simulink model "cm_test"  (R2015a)
settings: Solver=ode45  StartTime=0.0  StopTime=inf  MaxStep=1e-3  RelTol=1e-3
values from neighbouring files (symbols this model uses):
  ctr_law = struct    [Parameters.m]
  IMU = struct    [Parameters.m]
  lateral_control = true    [Parameters.m]
  longit_control = true    [Parameters.m]
  low_ctr = struct    [Parameters.m]
  mag = struct    [Parameters.m]
  steer_flag = 0    [Parameters.m]
  steer_sensor = struct    [Parameters.m]
  vhcl = struct    [Parameters.m]
undefined symbols (not defined in the file or in its folder): odo
libraries: CarMaker4SL x29, dspquant2 x6, simulink x1, aerolibtransform2 x1
(part 2 of 2)

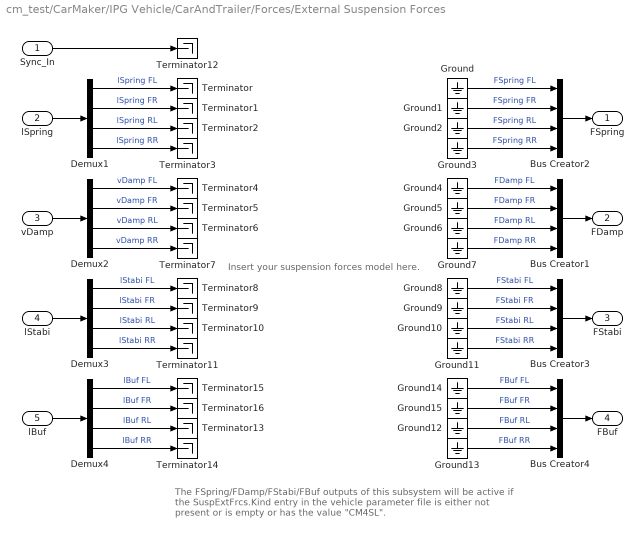
== system cm_test/CarMaker/IPG Vehicle/CarAndTrailer/Forces/External Suspension Forces ==
  note: The FSpring/FDamp/FStabi/FBuf outputs of this subsystem will be
      | active if the SuspExtFrcs.Kind entry in the vehicle parameter file
      | is either not present or is empty or has the value "CM4SL".
  note: Insert your suspension forces model here.
  Sync_In : Inport
  lSpring : Inport  Port=2
  vDamp : Inport  Port=3
  lStabi : Inport  Port=4
  lBuf : Inport  Port=5
  Bus Creator{1..4} (4 alike) : BusCreator
  Demux{1..4} (4 alike) : Demux
  Ground{,1..15} (16 alike) : Ground
  Terminator{,1..16} (17 alike) : Terminator
  FSpring : Outport
  FDamp : Outport  Port=2
  FStabi : Outport  Port=3
  FBuf : Outport  Port=4
  wires:
  lBuf/1 -> Demux4/1
  Demux4/1 -> Terminator15/1  "lBuf FL"
  Demux4/2 -> Terminator16/1  "lBuf FR"
  Demux4/3 -> Terminator13/1  "lBuf RL"
  Demux4/4 -> Terminator14/1  "lBuf RR"
  Ground14/1 -> Bus Creator4/1  "FBuf FL"
  Ground15/1 -> Bus Creator4/2  "FBuf FR"
  Ground12/1 -> Bus Creator4/3  "FBuf RL"
  Ground13/1 -> Bus Creator4/4  "FBuf RR"
  Bus Creator4/1 -> FBuf/1
  Sync_In/1 -> Terminator12/1
  lSpring/1 -> Demux1/1
  vDamp/1 -> Demux2/1
  lStabi/1 -> Demux3/1
  Demux3/1 -> Terminator8/1  "lStabi FL"
  Demux3/2 -> Terminator9/1  "lStabi FR"
  Demux3/3 -> Terminator10/1  "lStabi RL"
  Demux3/4 -> Terminator11/1  "lStabi RR"
  Demux1/1 -> Terminator/1  "lSpring FL"
  Demux1/2 -> Terminator1/1  "lSpring FR"
  Demux1/3 -> Terminator2/1  "lSpring RL"
  Demux1/4 -> Terminator3/1  "lSpring RR"
  Demux2/1 -> Terminator4/1  "vDamp FL"
  Demux2/2 -> Terminator5/1  "vDamp FR"
  Demux2/3 -> Terminator6/1  "vDamp RL"
  Demux2/4 -> Terminator7/1  "vDamp RR"
  Bus Creator2/1 -> FSpring/1
  Ground/1 -> Bus Creator2/1  "FSpring FL"
  Ground1/1 -> Bus Creator2/2  "FSpring FR"
  Ground2/1 -> Bus Creator2/3  "FSpring RL"
  Ground3/1 -> Bus Creator2/4  "FSpring RR"
  Ground4/1 -> Bus Creator1/1  "FDamp FL"
  Ground5/1 -> Bus Creator1/2  "FDamp FR"
  Ground6/1 -> Bus Creator1/3  "FDamp RL"
  Ground7/1 -> Bus Creator1/4  "FDamp RR"
  Bus Creator1/1 -> FDamp/1
  Ground8/1 -> Bus Creator3/1  "FStabi FL"
  Ground9/1 -> Bus Creator3/2  "FStabi FR"
  Ground10/1 -> Bus Creator3/3  "FStabi RL"
  Ground11/1 -> Bus Creator3/4  "FStabi RR"
  Bus Creator3/1 -> FStabi/1

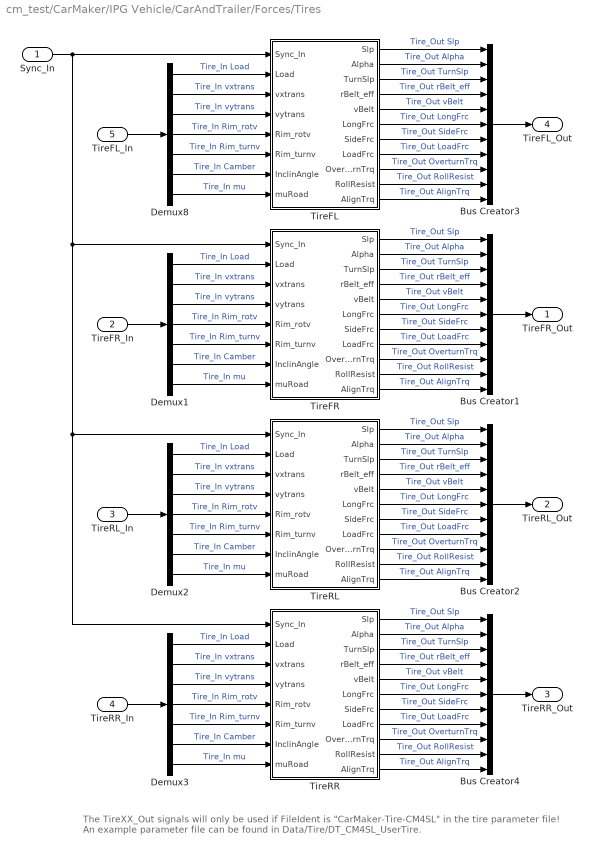
== system cm_test/CarMaker/IPG Vehicle/CarAndTrailer/Forces/Tires ==
  note: The TireXX_Out signals will only be used if FileIdent is "CarMaker-Tire-CM4SL" in the tire parameter file!
      | An example parameter file can be found in Data/Tire/DT_CM4SL_UserTire.
  Sync_In : Inport
  TireFR_In : Inport  Port=2
  TireRL_In : Inport  Port=3
  TireRR_In : Inport  Port=4
  TireFL_In : Inport  Port=5
  Bus Creator{1..4} (4 alike) : BusCreator  Inputs=11
  Demux{1..3,8} (4 alike) : Demux  Outputs=7
  TireFL : Subsystem
  TireFR : Subsystem
  TireRL : Subsystem
  TireRR : Subsystem
  TireFR_Out : Outport
  TireRL_Out : Outport  Port=2
  TireRR_Out : Outport  Port=3
  TireFL_Out : Outport  Port=4
  wires:
  Sync_In/1 -> TireRR/1(Sync_In), TireRL/1(Sync_In), TireFR/1(Sync_In), TireFL/1(Sync_In)
  Bus Creator4/1 -> TireRR_Out/1
  Bus Creator2/1 -> TireRL_Out/1
  Bus Creator1/1 -> TireFR_Out/1
  Demux3/5 -> TireRR/6(Rim_turnv)  "Tire_In Rim_turnv"
  Demux3/4 -> TireRR/5(Rim_rotv)  "Tire_In Rim_rotv"
  Demux3/1 -> TireRR/2(Load)  "Tire_In Load"
  Demux3/7 -> TireRR/8(muRoad)  "Tire_In mu"
  Demux3/6 -> TireRR/7(InclinAngle)  "Tire_In Camber"
  Demux3/2 -> TireRR/3(vxtrans)  "Tire_In vxtrans"
  Demux3/3 -> TireRR/4(vytrans)  "Tire_In vytrans"
  TireRR/11(AlignTrq) -> Bus Creator4/11  "Tire_Out AlignTrq"
  TireRR/10(RollResist) -> Bus Creator4/10  "Tire_Out RollResist"
  TireRR/9(OverturnTrq) -> Bus Creator4/9  "Tire_Out OverturnTrq"
  TireRR/8(LoadFrc) -> Bus Creator4/8  "Tire_Out LoadFrc"
  TireRR/7(SideFrc) -> Bus Creator4/7  "Tire_Out SideFrc"
  TireRR/6(LongFrc) -> Bus Creator4/6  "Tire_Out LongFrc"
  TireRR/5(vBelt) -> Bus Creator4/5  "Tire_Out vBelt"
  TireRR/4(rBelt_eff) -> Bus Creator4/4  "Tire_Out rBelt_eff"
  TireRR/3(TurnSlp) -> Bus Creator4/3  "Tire_Out TurnSlp"
  TireRR/1(Slp) -> Bus Creator4/1  "Tire_Out Slp"
  TireRR/2(Alpha) -> Bus Creator4/2  "Tire_Out Alpha"
  Demux2/5 -> TireRL/6(Rim_turnv)  "Tire_In Rim_turnv"
  Demux2/4 -> TireRL/5(Rim_rotv)  "Tire_In Rim_rotv"
  Demux2/1 -> TireRL/2(Load)  "Tire_In Load"
  Demux2/7 -> TireRL/8(muRoad)  "Tire_In mu"
  Demux2/6 -> TireRL/7(InclinAngle)  "Tire_In Camber"
  Demux2/2 -> TireRL/3(vxtrans)  "Tire_In vxtrans"
  Demux2/3 -> TireRL/4(vytrans)  "Tire_In vytrans"
  TireRL/11(AlignTrq) -> Bus Creator2/11  "Tire_Out AlignTrq"
  TireRL/10(RollResist) -> Bus Creator2/10  "Tire_Out RollResist"
  TireRL/9(OverturnTrq) -> Bus Creator2/9  "Tire_Out OverturnTrq"
  TireRL/8(LoadFrc) -> Bus Creator2/8  "Tire_Out LoadFrc"
  TireRL/7(SideFrc) -> Bus Creator2/7  "Tire_Out SideFrc"
  TireRL/6(LongFrc) -> Bus Creator2/6  "Tire_Out LongFrc"
  TireRL/5(vBelt) -> Bus Creator2/5  "Tire_Out vBelt"
  TireRL/4(rBelt_eff) -> Bus Creator2/4  "Tire_Out rBelt_eff"
  TireRL/3(TurnSlp) -> Bus Creator2/3  "Tire_Out TurnSlp"
  TireRL/1(Slp) -> Bus Creator2/1  "Tire_Out Slp"
  TireRL/2(Alpha) -> Bus Creator2/2  "Tire_Out Alpha"
  Demux1/5 -> TireFR/6(Rim_turnv)  "Tire_In Rim_turnv"
  Demux1/4 -> TireFR/5(Rim_rotv)  "Tire_In Rim_rotv"
  Demux1/1 -> TireFR/2(Load)  "Tire_In Load"
  Demux1/7 -> TireFR/8(muRoad)  "Tire_In mu"
  Demux1/6 -> TireFR/7(InclinAngle)  "Tire_In Camber"
  Demux1/2 -> TireFR/3(vxtrans)  "Tire_In vxtrans"
  Demux1/3 -> TireFR/4(vytrans)  "Tire_In vytrans"
  TireFR/11(AlignTrq) -> Bus Creator1/11  "Tire_Out AlignTrq"
  TireFR/10(RollResist) -> Bus Creator1/10  "Tire_Out RollResist"
  TireFR/9(OverturnTrq) -> Bus Creator1/9  "Tire_Out OverturnTrq"
  TireFR/8(LoadFrc) -> Bus Creator1/8  "Tire_Out LoadFrc"
  TireFR/7(SideFrc) -> Bus Creator1/7  "Tire_Out SideFrc"
  TireFR/6(LongFrc) -> Bus Creator1/6  "Tire_Out LongFrc"
  TireFR/5(vBelt) -> Bus Creator1/5  "Tire_Out vBelt"
  TireFR/4(rBelt_eff) -> Bus Creator1/4  "Tire_Out rBelt_eff"
  TireFR/3(TurnSlp) -> Bus Creator1/3  "Tire_Out TurnSlp"
  TireFR/1(Slp) -> Bus Creator1/1  "Tire_Out Slp"
  TireFR/2(Alpha) -> Bus Creator1/2  "Tire_Out Alpha"
  Demux8/5 -> TireFL/6(Rim_turnv)  "Tire_In Rim_turnv"
  Demux8/4 -> TireFL/5(Rim_rotv)  "Tire_In Rim_rotv"
  TireFL_In/1 -> Demux8/1
  Demux8/1 -> TireFL/2(Load)  "Tire_In Load"
  Demux8/7 -> TireFL/8(muRoad)  "Tire_In mu"
  Demux8/6 -> TireFL/7(InclinAngle)  "Tire_In Camber"
  Demux8/2 -> TireFL/3(vxtrans)  "Tire_In vxtrans"
  Demux8/3 -> TireFL/4(vytrans)  "Tire_In vytrans"
  TireFL/11(AlignTrq) -> Bus Creator3/11  "Tire_Out AlignTrq"
  TireFL/10(RollResist) -> Bus Creator3/10  "Tire_Out RollResist"
  TireFL/9(OverturnTrq) -> Bus Creator3/9  "Tire_Out OverturnTrq"
  TireFL/8(LoadFrc) -> Bus Creator3/8  "Tire_Out LoadFrc"
  TireFL/7(SideFrc) -> Bus Creator3/7  "Tire_Out SideFrc"
  TireFL/6(LongFrc) -> Bus Creator3/6  "Tire_Out LongFrc"
  TireFL/5(vBelt) -> Bus Creator3/5  "Tire_Out vBelt"
  TireFL/4(rBelt_eff) -> Bus Creator3/4  "Tire_Out rBelt_eff"
  TireFL/3(TurnSlp) -> Bus Creator3/3  "Tire_Out TurnSlp"
  TireFL/1(Slp) -> Bus Creator3/1  "Tire_Out Slp"
  TireFL/2(Alpha) -> Bus Creator3/2  "Tire_Out Alpha"
  Bus Creator3/1 -> TireFL_Out/1
  TireFR_In/1 -> Demux1/1
  TireRL_In/1 -> Demux2/1
  TireRR_In/1 -> Demux3/1

== system cm_test/CarMaker/IPG Vehicle/CarAndTrailer/Forces/Vehicle Forces ==
  Sync_In : Inport
  Bus Creator1 : BusCreator  Inputs=12
  Bus Creator5 : BusCreator  Inputs=13
  Bus Creator8 : BusCreator  Inputs=16
  Demux : Demux  Outputs=16
  Demux1 : Demux  Outputs=12
  Demux5 : Demux  Outputs=13
  Forces : S-Function  FunctionName=CM_Sfun  Parameters='Forces'
  Sync_Out : Outport
  Car.Virtual : Outport  Port=2
  Car.Aero : Outport  Port=3
  Car.Load : Outport  Port=4
  wires:
  Demux/16 -> Bus Creator8/16  "Car Load_3 tz"
  Demux/15 -> Bus Creator8/15  "Car Load_3 ty"
  Demux/14 -> Bus Creator8/14  "Car Load_3 tx"
  Demux/13 -> Bus Creator8/13  "Car Load_3 mass"
  Demux1/12 -> Bus Creator1/12  "Car Virtual Trq_0 z"
  Demux1/11 -> Bus Creator1/11  "Car Virtual Trq_0 y"
  Demux1/10 -> Bus Creator1/10  "Car Virtual Trq_0 x"
  Demux1/9 -> Bus Creator1/9  "Car Virtual Trq_1 z"
  Demux1/8 -> Bus Creator1/8  "Car Virtual Trq_1 y"
  Demux1/7 -> Bus Creator1/7  "Car Virtual Trq_1 x"
  Demux1/6 -> Bus Creator1/6  "Car Virtual Frc_0 z"
  Demux1/5 -> Bus Creator1/5  "Car Virtual Frc_0 y"
  Demux1/4 -> Bus Creator1/4  "Car Virtual Frc_0 x"
  Sync_In/1 -> Forces/1
  Forces/1 -> Sync_Out/1
  Bus Creator5/1 -> Car.Aero/1
  Demux1/1 -> Bus Creator1/1  "Car Virtual Frc_1 x"
  Demux1/2 -> Bus Creator1/2  "Car Virtual Frc_1 y"
  Demux1/3 -> Bus Creator1/3  "Car Virtual Frc_1 z"
  Forces/3 -> Demux5/1
  Forces/2 -> Demux1/1
  Bus Creator1/1 -> Car.Virtual/1
  Bus Creator8/1 -> Car.Load/1
  Demux/1 -> Bus Creator8/1  "Car Load_0 mass"
  Demux/2 -> Bus Creator8/2  "Car Load_0 tx"
  Demux/3 -> Bus Creator8/3  "Car Load_0 ty"
  Demux/4 -> Bus Creator8/4  "Car Load_0 tz"
  Demux/5 -> Bus Creator8/5  "Car Load_1 mass"
  Demux/6 -> Bus Creator8/6  "Car Load_1 tx"
  Demux/7 -> Bus Creator8/7  "Car Load_1 ty"
  Demux/8 -> Bus Creator8/8  "Car Load_1 tz"
  Demux/9 -> Bus Creator8/9  "Car Load_2 mass"
  Demux/10 -> Bus Creator8/10  "Car Load_2 tx"
  Demux/11 -> Bus Creator8/11  "Car Load_2 ty"
  Demux/12 -> Bus Creator8/12  "Car Load_2 tz"
  Forces/4 -> Demux/1
  Demux5/11 -> Bus Creator5/11  "car Aero Trq_1 x"
  Demux5/12 -> Bus Creator5/12  "car Aero Trq_1 y"
  Demux5/13 -> Bus Creator5/13  "car Aero Trq_1 z"
  Demux5/10 -> Bus Creator5/10  "car Aero Frc_1 z"
  Demux5/9 -> Bus Creator5/9  "car Aero Frc_1 y"
  Demux5/8 -> Bus Creator5/8  "car Aero Frc_1 x"
  Demux5/1 -> Bus Creator5/1  "Vehicle sRoadAero"
  Demux5/2 -> Bus Creator5/2  "Vehicle Wind_vel_0 x"
  Demux5/3 -> Bus Creator5/3  "Vehicle Wind_vel_0 y"
  Demux5/4 -> Bus Creator5/4  "Vehicle Wind_vel_0 z"
  Demux5/5 -> Bus Creator5/5  "car Aero vRes_1 x"
  Demux5/6 -> Bus Creator5/6  "car Aero vRes_1 y"
  Demux5/7 -> Bus Creator5/7  "car Aero vRes_1 z"

== system cm_test/CarMaker/IPG Vehicle/CarAndTrailer/Trailer/CreateBus Car.Hitch.FrcTrq ==
  In1 : Inport
  Bus Creator7 : BusCreator  Inputs=6
  Demux7 : Demux  Outputs=6
  Car.Hitch.FrcTrq : Outport
  wires:
  In1/1 -> Demux7/1
  Bus Creator7/1 -> Car.Hitch.FrcTrq/1
  Demux7/6 -> Bus Creator7/6  "Car Hitch Trq2Car z"
  Demux7/5 -> Bus Creator7/5  "Car Hitch Trq2Car y"
  Demux7/4 -> Bus Creator7/4  "Car Hitch Trq2Car x"
  Demux7/3 -> Bus Creator7/3  "Car Hitch Frc2Car z"
  Demux7/2 -> Bus Creator7/2  "Car Hitch Frc2Car y"
  Demux7/1 -> Bus Creator7/1  "Car Hitch Frc2Car x"

== system cm_test/CarMaker/IPG Vehicle/CarAndTrailer/Trailer/CreateBus Vhcl.Motion ==
  In1 : Inport
  Demux1 : Demux  Outputs=16
  Mux1 : Mux  Inputs=16
  Out1 : Outport
  wires:
  Demux1/1 -> Mux1/1  "Vhcl v"
  Demux1/2 -> Mux1/2  "Vhcl Distance"
  Demux1/3 -> Mux1/3  "Vhcl sRoad"
  Demux1/4 -> Mux1/4  "Vhcl sRoadAero"
  Demux1/5 -> Mux1/5  "Vhcl Hitch_Pos x"
  Demux1/6 -> Mux1/6  "Vhcl Hitch_Pos y"
  Demux1/7 -> Mux1/7  "Vhcl Hitch_Pos z"
  Demux1/8 -> Mux1/8  "Vhcl Roll"
  Demux1/9 -> Mux1/9  "Vhcl RollVel"
  Demux1/10 -> Mux1/10  "Vhcl RollAcc"
  Demux1/11 -> Mux1/11  "Vhcl Pitch"
  Demux1/12 -> Mux1/12  "Vhcl PitchVel"
  Demux1/13 -> Mux1/13  "Vhcl PitchAcc"
  Demux1/14 -> Mux1/14  "Vhcl Yaw"
  Demux1/15 -> Mux1/15  "Vhcl YawRate"
  Demux1/16 -> Mux1/16  "Vhcl YawAcc"
  In1/1 -> Demux1/1
  Mux1/1 -> Out1/1

== system cm_test/CarMaker/IPG Vehicle/CarAndTrailer/Trailer/CreateBus Vhcl.PoI ==
  In1 : Inport
  Bus Creator3 : BusCreator  Inputs=18
  Demux3 : Demux  Outputs=18
  Out1 : Outport
  wires:
  Demux3/18 -> Bus Creator3/18  "Vhcl PoI_GCS Elev"
  Demux3/17 -> Bus Creator3/17  "Vhcl PoI_GCS Lat"
  Demux3/16 -> Bus Creator3/16  "Vhcl PoI_GCS Long"
  Demux3/15 -> Bus Creator3/15  "Vhcl PoI_Acc_1 z"
  Demux3/14 -> Bus Creator3/14  "Vhcl PoI_Acc_1 y"
  Demux3/13 -> Bus Creator3/13  "Vhcl PoI_Acc_1 x"
  Demux3/12 -> Bus Creator3/12  "Vhcl PoI_Vel_1 z"
  Demux3/11 -> Bus Creator3/11  "Vhcl PoI_Vel_1 y"
  Demux3/10 -> Bus Creator3/10  "Vhcl PoI_Vel_1 x"
  Demux3/9 -> Bus Creator3/9  "Vhcl PoI_Acc z"
  Demux3/8 -> Bus Creator3/8  "Vhcl PoI_Acc y"
  Demux3/7 -> Bus Creator3/7  "Vhcl PoI_Acc x"
  Demux3/6 -> Bus Creator3/6  "Vhcl PoI_Vel z"
  Demux3/5 -> Bus Creator3/5  "Vhcl PoI_Vel y"
  Demux3/4 -> Bus Creator3/4  "Vhcl PoI_Vel x"
  Demux3/3 -> Bus Creator3/3  "Vhcl PoI_Pos z"
  Demux3/2 -> Bus Creator3/2  "Vhcl PoI_Pos y"
  In1/1 -> Demux3/1
  Bus Creator3/1 -> Out1/1
  Demux3/1 -> Bus Creator3/1  "Vhcl PoI_Pos x"

== system cm_test/CarMaker/IPG Vehicle/CarAndTrailer/Trailer/CreateBus Vhcl.Steering ==
  In1 : Inport
  Bus Creator3 : BusCreator
  Demux : Demux
  Out1 : Outport
  wires:
  Bus Creator3/1 -> Out1/1
  Demux/1 -> Bus Creator3/1  "Vhcl Steering Ang"
  Demux/3 -> Bus Creator3/3  "Vhcl Steering AngAcc"
  Demux/2 -> Bus Creator3/2  "Vhcl Steering AngVel"
  Demux/4 -> Bus Creator3/4  "Vhcl Steering Trq"
  In1/1 -> Demux/1

== system cm_test/CarMaker/IPG Vehicle/CarAndTrailer/Trailer/CreateBus Vhcl.Wheel.FL ==
  In1 : Inport
  Bus Creator3 : BusCreator  Inputs=14
  Demux3 : Demux  Outputs=14
  Out1 : Outport
  wires:
  Demux3/14 -> Bus Creator3/14  "Vhcl Wheel FL Trq_WhlBearing"
  Demux3/13 -> Bus Creator3/13  "Vhcl Wheel FL Trq_T2W"
  Demux3/12 -> Bus Creator3/12  "Vhcl Wheel FL SideSlip"
  Demux3/11 -> Bus Creator3/11  "Vhcl Wheel FL LongSlip"
  Demux3/10 -> Bus Creator3/10  "Vhcl Wheel FL vBelt"
  Demux3/9 -> Bus Creator3/9  "Vhcl Wheel FL Fz"
  Demux3/8 -> Bus Creator3/8  "Vhcl Wheel FL Fy"
  Demux3/7 -> Bus Creator3/7  "Vhcl Wheel FL Fx"
  Demux3/6 -> Bus Creator3/6  "Vhcl Wheel FL r_zxy z"
  Demux3/5 -> Bus Creator3/5  "Vhcl Wheel FL r_zxy y"
  Demux3/4 -> Bus Creator3/4  "Vhcl Wheel FL r_zxy x"
  Demux3/3 -> Bus Creator3/3  "Vhcl Wheel FL t z"
  Demux3/2 -> Bus Creator3/2  "Vhcl Wheel FL t y"
  In1/1 -> Demux3/1
  Bus Creator3/1 -> Out1/1
  Demux3/1 -> Bus Creator3/1  "Vhcl Wheel FL t x"

== system cm_test/CarMaker/IPG Vehicle/CarAndTrailer/Trailer/CreateBus Vhcl.Wheel.FR ==
  In1 : Inport
  Bus Creator3 : BusCreator  Inputs=14
  Demux3 : Demux  Outputs=14
  Out1 : Outport
  wires:
  Demux3/14 -> Bus Creator3/14  "Vhcl Wheel FR Trq_WhlBearing"
  Demux3/13 -> Bus Creator3/13  "Vhcl Wheel FR Trq_T2W"
  Demux3/12 -> Bus Creator3/12  "Vhcl Wheel FR SideSlip"
  Demux3/11 -> Bus Creator3/11  "Vhcl Wheel FR LongSlip"
  Demux3/10 -> Bus Creator3/10  "Vhcl Wheel FR vBelt"
  Demux3/9 -> Bus Creator3/9  "Vhcl Wheel FR Fz"
  Demux3/8 -> Bus Creator3/8  "Vhcl Wheel FR Fy"
  Demux3/7 -> Bus Creator3/7  "Vhcl Wheel FR Fx"
  Demux3/6 -> Bus Creator3/6  "Vhcl Wheel FR r_zxy z"
  Demux3/5 -> Bus Creator3/5  "Vhcl Wheel FR r_zxy y"
  Demux3/4 -> Bus Creator3/4  "Vhcl Wheel FR r_zxy x"
  Demux3/3 -> Bus Creator3/3  "Vhcl Wheel FR t z"
  Demux3/2 -> Bus Creator3/2  "Vhcl Wheel FR t y"
  In1/1 -> Demux3/1
  Bus Creator3/1 -> Out1/1
  Demux3/1 -> Bus Creator3/1  "Vhcl Wheel FR t x"

== system cm_test/CarMaker/IPG Vehicle/CarAndTrailer/Trailer/CreateBus Vhcl.Wheel.RL ==
  In1 : Inport
  Bus Creator3 : BusCreator  Inputs=14
  Demux3 : Demux  Outputs=14
  Out1 : Outport
  wires:
  Demux3/14 -> Bus Creator3/14  "Vhcl Wheel RL Trq_WhlBearing"
  Demux3/13 -> Bus Creator3/13  "Vhcl Wheel RL Trq_T2W"
  Demux3/12 -> Bus Creator3/12  "Vhcl Wheel RL SideSlip"
  Demux3/11 -> Bus Creator3/11  "Vhcl Wheel RL LongSlip"
  Demux3/10 -> Bus Creator3/10  "Vhcl Wheel RL vBelt"
  Demux3/9 -> Bus Creator3/9  "Vhcl Wheel RL Fz"
  Demux3/8 -> Bus Creator3/8  "Vhcl Wheel RL Fy"
  Demux3/7 -> Bus Creator3/7  "Vhcl Wheel RL Fx"
  Demux3/6 -> Bus Creator3/6  "Vhcl Wheel RL r_zxy z"
  Demux3/5 -> Bus Creator3/5  "Vhcl Wheel RL r_zxy y"
  Demux3/4 -> Bus Creator3/4  "Vhcl Wheel RL r_zxy x"
  Demux3/3 -> Bus Creator3/3  "Vhcl Wheel RL t z"
  Demux3/2 -> Bus Creator3/2  "Vhcl Wheel RL t y"
  In1/1 -> Demux3/1
  Bus Creator3/1 -> Out1/1
  Demux3/1 -> Bus Creator3/1  "Vhcl Wheel RL t x"

== system cm_test/CarMaker/IPG Vehicle/CarAndTrailer/Trailer/CreateBus Vhcl.Wheel.RR ==
  In1 : Inport
  Bus Creator3 : BusCreator  Inputs=14
  Demux3 : Demux  Outputs=14
  Out1 : Outport
  wires:
  Demux3/14 -> Bus Creator3/14  "Vhcl Wheel RR Trq_WhlBearing"
  Demux3/13 -> Bus Creator3/13  "Vhcl Wheel RR Trq_T2W"
  Demux3/12 -> Bus Creator3/12  "Vhcl Wheel RR SideSlip"
  Demux3/11 -> Bus Creator3/11  "Vhcl Wheel RR LongSlip"
  Demux3/10 -> Bus Creator3/10  "Vhcl Wheel RR vBelt"
  Demux3/9 -> Bus Creator3/9  "Vhcl Wheel RR Fz"
  Demux3/8 -> Bus Creator3/8  "Vhcl Wheel RR Fy"
  Demux3/7 -> Bus Creator3/7  "Vhcl Wheel RR Fx"
  Demux3/6 -> Bus Creator3/6  "Vhcl Wheel RR r_zxy z"
  Demux3/5 -> Bus Creator3/5  "Vhcl Wheel RR r_zxy y"
  Demux3/4 -> Bus Creator3/4  "Vhcl Wheel RR r_zxy x"
  Demux3/3 -> Bus Creator3/3  "Vhcl Wheel RR t z"
  Demux3/2 -> Bus Creator3/2  "Vhcl Wheel RR t y"
  In1/1 -> Demux3/1
  Bus Creator3/1 -> Out1/1
  Demux3/1 -> Bus Creator3/1  "Vhcl Wheel RR t x"

== system cm_test/CarMaker/VehicleControl/Sensors/IMU/Accelerometers ==
  Mux : Mux  Inputs=3
  Read Alpha.x : CarMaker4SL/Read CM Dict  xname=BodySensor.BD00.Alpha_0.x  xsync=off
  Read Alpha.y : CarMaker4SL/Read CM Dict  xname=BodySensor.BD00.Alpha_0.y  xsync=off
  Read Alpha.z : CarMaker4SL/Read CM Dict  xname=BodySensor.BD00.Alpha_0.z  xsync=off
  Scope : Scope
  Scope1 : Scope
  Scope2 : Scope
  accels_out : Outport
  wires:
  Read Alpha.y/1 -> Scope1/1, Mux/2
  Read Alpha.x/1 -> Scope/1, Mux/1
  Read Alpha.z/1 -> Scope2/1, Mux/3
  Mux/1 -> accels_out/1

== system cm_test/CarMaker/VehicleControl/Sensors/IMU/Gyroscopes ==
  Mux : Mux  Inputs=3
  Read Omega.x : CarMaker4SL/Read CM Dict  xname=BodySensor.BD00.Omega_0.x  xsync=off
  Read Omega.y : CarMaker4SL/Read CM Dict  xname=BodySensor.BD00.Omega_0.y  xsync=off
  Read Omega.z : CarMaker4SL/Read CM Dict  xname=BodySensor.BD00.Omega_0.z  xsync=off
  Scope : Scope
      settings: YMin=-10  YMax=10
  Scope1 : Scope
  Scope2 : Scope
  gyros_out : Outport
  wires:
  Read Omega.y/1 -> Scope1/1, Mux/2
  Read Omega.x/1 -> Scope/1, Mux/1
  Read Omega.z/1 -> Scope2/1, Mux/3
  Mux/1 -> gyros_out/1

== system cm_test/CarMaker/VehicleControl/Sensors/RPSensor/Preview pt pos in Fr1 ==
  Display{,1..3} (4 alike) : Display
  MatProduct : Product  Multiplication=Matrix(*)
  Rotation Angles to Direction Cosine Matrix : aerolibtransform2/Rotation Angles to Direction Cosine Matrix  rotationOrder=ZYX
  car rotation in Fr0 : Subsystem
  preview pt pos in Fr0 with car origin as origin of Fr0 : Subsystem
  prev_pt_pos_Fr1 : Outport
  wires:
  Rotation Angles to Direction Cosine Matrix/1 -> Display1/1, MatProduct/1
  preview pt pos in Fr0 with car origin as origin of Fr0/1(prev_pt_pos_Fr0) -> Display3/1, MatProduct/2  "prev_pt_pos_Fr0"
  car rotation in Fr0/1(3D_angle) -> Display/1, Rotation Angles to Direction Cosine Matrix/1
  MatProduct/1 -> Display2/1, prev_pt_pos_Fr1/1  "prev_pt_pos_Fr1"

== system cm_test/CarMaker/VehicleControl/Sensors/Steering angle (rad)/Mean of 2 values ==
  vec : Inport
  Add : Sum
  Demux : Demux  Outputs=2
  Gain : Gain  Gain=0.5
  mean : Outport
  wires:
  Add/1 -> Gain/1
  Gain/1 -> mean/1
  Demux/2 -> Add/2
  Demux/1 -> Add/1
  vec/1 -> Demux/1

== system cm_test/CarMaker/VehicleControl/Sensors/odometry/Mean of 2 values ==
  vec : Inport
  Add : Sum
  Demux : Demux  Outputs=2
  Gain : Gain  Gain=0.5
  mean : Outport
  wires:
  Add/1 -> Gain/1
  Gain/1 -> mean/1
  Demux/2 -> Add/2
  Demux/1 -> Add/1
  vec/1 -> Demux/1

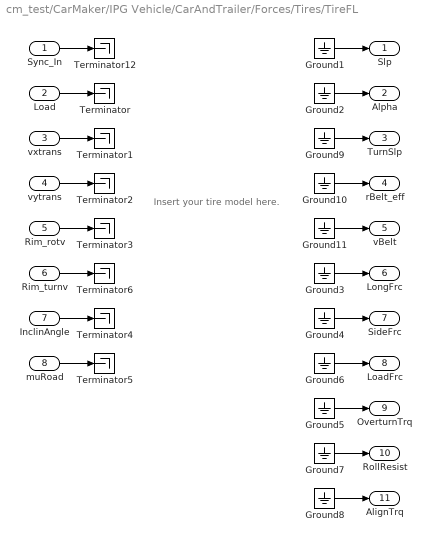
== system cm_test/CarMaker/IPG Vehicle/CarAndTrailer/Forces/Tires/TireFL ==
  note: Insert your tire model here.
  Sync_In : Inport
  Load : Inport  Port=2
  vxtrans : Inport  Port=3
  vytrans : Inport  Port=4
  Rim_rotv : Inport  Port=5
  Rim_turnv : Inport  Port=6
  InclinAngle : Inport  Port=7
  muRoad : Inport  Port=8
  Ground{1..11} (11 alike) : Ground
  Terminator{,1..6,12} (8 alike) : Terminator
  Slp : Outport
  Alpha : Outport  Port=2
  TurnSlp : Outport  Port=3
  rBelt_eff : Outport  Port=4
  vBelt : Outport  Port=5
  LongFrc : Outport  Port=6
  SideFrc : Outport  Port=7
  LoadFrc : Outport  Port=8
  OverturnTrq : Outport  Port=9
  RollResist : Outport  Port=10
  AlignTrq : Outport  Port=11
  wires:
  Ground11/1 -> vBelt/1
  Ground10/1 -> rBelt_eff/1
  Ground9/1 -> TurnSlp/1
  Rim_turnv/1 -> Terminator6/1
  Sync_In/1 -> Terminator12/1
  Ground2/1 -> Alpha/1
  Ground3/1 -> LongFrc/1
  Ground4/1 -> SideFrc/1
  Ground5/1 -> OverturnTrq/1
  vxtrans/1 -> Terminator1/1
  vytrans/1 -> Terminator2/1
  Rim_rotv/1 -> Terminator3/1
  InclinAngle/1 -> Terminator4/1
  muRoad/1 -> Terminator5/1
  Load/1 -> Terminator/1
  Ground1/1 -> Slp/1
  Ground6/1 -> LoadFrc/1
  Ground7/1 -> RollResist/1
  Ground8/1 -> AlignTrq/1

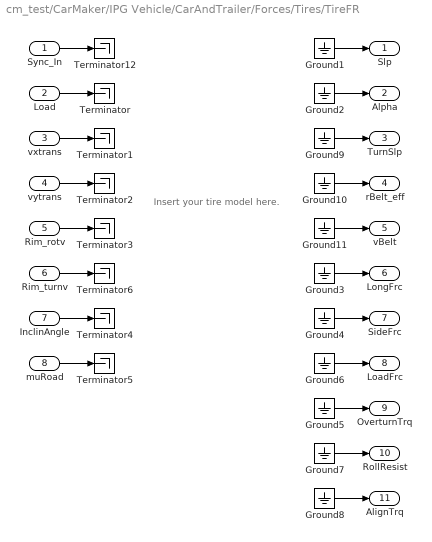
== system cm_test/CarMaker/IPG Vehicle/CarAndTrailer/Forces/Tires/TireFR ==
  note: Insert your tire model here.
  Sync_In : Inport
  Load : Inport  Port=2
  vxtrans : Inport  Port=3
  vytrans : Inport  Port=4
  Rim_rotv : Inport  Port=5
  Rim_turnv : Inport  Port=6
  InclinAngle : Inport  Port=7
  muRoad : Inport  Port=8
  Ground{1..11} (11 alike) : Ground
  Terminator{,1..6,12} (8 alike) : Terminator
  Slp : Outport
  Alpha : Outport  Port=2
  TurnSlp : Outport  Port=3
  rBelt_eff : Outport  Port=4
  vBelt : Outport  Port=5
  LongFrc : Outport  Port=6
  SideFrc : Outport  Port=7
  LoadFrc : Outport  Port=8
  OverturnTrq : Outport  Port=9
  RollResist : Outport  Port=10
  AlignTrq : Outport  Port=11
  wires:
  Ground11/1 -> vBelt/1
  Ground10/1 -> rBelt_eff/1
  Ground9/1 -> TurnSlp/1
  Rim_turnv/1 -> Terminator6/1
  Sync_In/1 -> Terminator12/1
  Ground2/1 -> Alpha/1
  Ground3/1 -> LongFrc/1
  Ground4/1 -> SideFrc/1
  Ground5/1 -> OverturnTrq/1
  vxtrans/1 -> Terminator1/1
  vytrans/1 -> Terminator2/1
  Rim_rotv/1 -> Terminator3/1
  InclinAngle/1 -> Terminator4/1
  muRoad/1 -> Terminator5/1
  Load/1 -> Terminator/1
  Ground1/1 -> Slp/1
  Ground6/1 -> LoadFrc/1
  Ground7/1 -> RollResist/1
  Ground8/1 -> AlignTrq/1

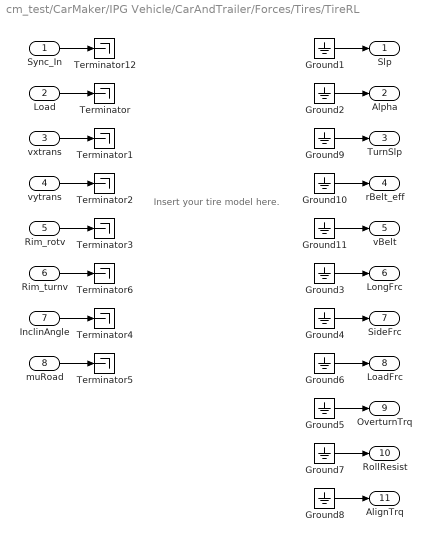
== system cm_test/CarMaker/IPG Vehicle/CarAndTrailer/Forces/Tires/TireRL ==
  note: Insert your tire model here.
  Sync_In : Inport
  Load : Inport  Port=2
  vxtrans : Inport  Port=3
  vytrans : Inport  Port=4
  Rim_rotv : Inport  Port=5
  Rim_turnv : Inport  Port=6
  InclinAngle : Inport  Port=7
  muRoad : Inport  Port=8
  Ground{1..11} (11 alike) : Ground
  Terminator{,1..6,12} (8 alike) : Terminator
  Slp : Outport
  Alpha : Outport  Port=2
  TurnSlp : Outport  Port=3
  rBelt_eff : Outport  Port=4
  vBelt : Outport  Port=5
  LongFrc : Outport  Port=6
  SideFrc : Outport  Port=7
  LoadFrc : Outport  Port=8
  OverturnTrq : Outport  Port=9
  RollResist : Outport  Port=10
  AlignTrq : Outport  Port=11
  wires:
  Ground11/1 -> vBelt/1
  Ground10/1 -> rBelt_eff/1
  Ground9/1 -> TurnSlp/1
  Rim_turnv/1 -> Terminator6/1
  Sync_In/1 -> Terminator12/1
  Ground2/1 -> Alpha/1
  Ground3/1 -> LongFrc/1
  Ground4/1 -> SideFrc/1
  Ground5/1 -> OverturnTrq/1
  vxtrans/1 -> Terminator1/1
  vytrans/1 -> Terminator2/1
  Rim_rotv/1 -> Terminator3/1
  InclinAngle/1 -> Terminator4/1
  muRoad/1 -> Terminator5/1
  Load/1 -> Terminator/1
  Ground1/1 -> Slp/1
  Ground6/1 -> LoadFrc/1
  Ground7/1 -> RollResist/1
  Ground8/1 -> AlignTrq/1

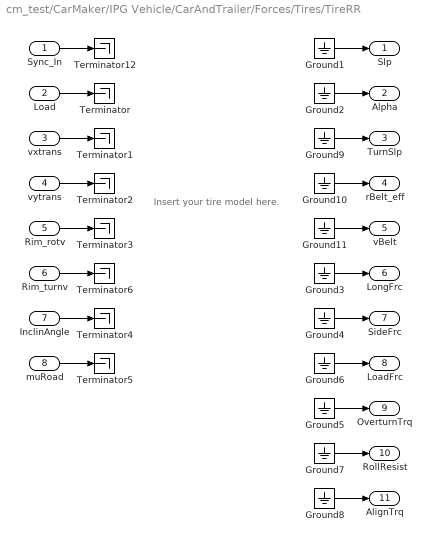
== system cm_test/CarMaker/IPG Vehicle/CarAndTrailer/Forces/Tires/TireRR ==
  note: Insert your tire model here.
  Sync_In : Inport
  Load : Inport  Port=2
  vxtrans : Inport  Port=3
  vytrans : Inport  Port=4
  Rim_rotv : Inport  Port=5
  Rim_turnv : Inport  Port=6
  InclinAngle : Inport  Port=7
  muRoad : Inport  Port=8
  Ground{1..11} (11 alike) : Ground
  Terminator{,1..6,12} (8 alike) : Terminator
  Slp : Outport
  Alpha : Outport  Port=2
  TurnSlp : Outport  Port=3
  rBelt_eff : Outport  Port=4
  vBelt : Outport  Port=5
  LongFrc : Outport  Port=6
  SideFrc : Outport  Port=7
  LoadFrc : Outport  Port=8
  OverturnTrq : Outport  Port=9
  RollResist : Outport  Port=10
  AlignTrq : Outport  Port=11
  wires:
  Ground11/1 -> vBelt/1
  Ground10/1 -> rBelt_eff/1
  Ground9/1 -> TurnSlp/1
  Rim_turnv/1 -> Terminator6/1
  Sync_In/1 -> Terminator12/1
  Ground2/1 -> Alpha/1
  Ground3/1 -> LongFrc/1
  Ground4/1 -> SideFrc/1
  Ground5/1 -> OverturnTrq/1
  vxtrans/1 -> Terminator1/1
  vytrans/1 -> Terminator2/1
  Rim_rotv/1 -> Terminator3/1
  InclinAngle/1 -> Terminator4/1
  muRoad/1 -> Terminator5/1
  Load/1 -> Terminator/1
  Ground1/1 -> Slp/1
  Ground6/1 -> LoadFrc/1
  Ground7/1 -> RollResist/1
  Ground8/1 -> AlignTrq/1

== system cm_test/CarMaker/VehicleControl/Sensors/RPSensor/Preview pt pos in Fr1/car rotation in Fr0 ==
  Mux : Mux  Inputs=3
  pitch angle : CarMaker4SL/Read CM Dict  xname=Vhcl.Pitch  xsync=off
  roll angle : CarMaker4SL/Read CM Dict  xname=Vhcl.Roll  xsync=off
  yaw angle : CarMaker4SL/Read CM Dict  xname=Vhcl.Yaw  xsync=off
  3D_angle : Outport
  wires:
  pitch angle/1 -> Mux/2
  roll angle/1 -> Mux/3
  yaw angle/1 -> Mux/1
  Mux/1 -> 3D_angle/1

== system cm_test/CarMaker/VehicleControl/Sensors/RPSensor/Preview pt pos in Fr1/preview pt pos in Fr0 with car origin as origin of Fr0 ==
  Display : Display
  Display1 : Display
  ground truth absolute pos of preview point : Subsystem
  ground truth absolute pos of vehicle origin (rear of vehicle) : Subsystem
  sub : Sum  Inputs=+-
  prev_pt_pos_Fr0 : Outport
  wires:
  sub/1 -> prev_pt_pos_Fr0/1
  ground truth absolute pos of vehicle origin (rear of vehicle)/1(vehicle_pos) -> Display1/1, sub/2
  ground truth absolute pos of preview point/1(preview_point_pos) -> Display/1, sub/1

== system cm_test/CarMaker/VehicleControl/Sensors/RPSensor/Preview pt pos in Fr1/preview pt pos in Fr0 with car origin as origin of Fr0/ground truth absolute pos of preview point ==
  Mux : Mux  Inputs=3
  Preview point absolute position : CarMaker4SL/Read CM Dict  xname=RPSensor.RP00.Path.tx  xsync=off
  Preview point absolute position1 : CarMaker4SL/Read CM Dict  xname=RPSensor.RP00.Path.ty  xsync=off
  Preview point absolute position2 : CarMaker4SL/Read CM Dict  xname=RPSensor.RP00.Path.tz  xsync=off
  preview_point_pos : Outport
  wires:
  Preview point absolute position/1 -> Mux/1
  Mux/1 -> preview_point_pos/1
  Preview point absolute position2/1 -> Mux/3
  Preview point absolute position1/1 -> Mux/2

== system cm_test/CarMaker/VehicleControl/Sensors/RPSensor/Preview pt pos in Fr1/preview pt pos in Fr0 with car origin as origin of Fr0/ground truth absolute pos of vehicle origin (rear of vehicle) ==
  Mux : Mux  Inputs=3
  Vehicle origin absolute position -x : CarMaker4SL/Read CM Dict  xname=Vhcl.Fr1.x  xsync=off
  Vehicle origin absolute position -y : CarMaker4SL/Read CM Dict  xname=Vhcl.Fr1.y  xsync=off
  Vehicle origin absolute position- z : CarMaker4SL/Read CM Dict  xname=Vhcl.Fr1.z  xsync=off
  vehicle_pos : Outport
  wires:
  Vehicle origin absolute position -x/1 -> Mux/1
  Vehicle origin absolute position -y/1 -> Mux/2
  Vehicle origin absolute position- z/1 -> Mux/3
  Mux/1 -> vehicle_pos/1

== matlab function cm_test/CarMaker/VehicleControl/Autonomous driving/low level controller ==
  data: sensors_in input; v_ref input; gamma_ref input; accel output; steer_flag input; low_ctr input; vhcl input; steer output
function [accel, steer] = fcn(sensors_in, v_ref, gamma_ref, steer_flag, ...
    low_ctr, vhcl)
%% Transforms output of control law into driver-like inputs for CM model
% implements low level controllers for steerign and speed and maps the
% outputs to be fed to CarMaker "VehicleControlUpd" model.
% 
% inputs:
% - target speed or acceleration
% - target steering angle (at front wheels)
%
% outputs:
% accel vector, composed of:
%   - brake
%   - gas
% steer vector composed of: 
%   - steering angle at steering wheel
%   - steering velocity at steering wheel
%   - steering accel at steering wheel
%   - steering torque at steering wheel
%
% depending on the steering mode, some of the steering signals might be set
% to zero.

%% Retrieves inputs and parameters

Fs = low_ctr.Fs;

% measures for feedback
% longitudinal acceleration
% a = sensors_in.imu_out.Alpha_0(1);
% actual speed
v = sensors_in.odo_out.vel_from_motor;

% wheel radius
R_wheel = vhcl.wheel_radius;

% vehicle mass
mass = vhcl.mass;

% mapping coeff for gas pedal (linear coeff only for the moment)
torque_to_gas = 1 ./ (low_ctr.trq_full - low_ctr.trq_zero);

% mapping for brake pedal
% vector of 2 coeffs: 1 for a front wheel and 1 for a rear wheel.
% to directly have the torque for an axle, the brake_to_Trq coeffs have
% been multiplied by 2.
torque_to_brake = 1 ./ (2*low_ctr.brake_to_Trq);

% steering angle to angle of steering wheel
steer_coeff = low_ctr.st_angle_to_st_wheel;

% CAREFUL: mappings for steering and brake are approximate. Need a proper
% control loop (along with smooth references) to ensure proper tracking.

%% Output initialization

steer_angle = 0;
steer_vel = 0;
steer_acc = 0;
steer_torque = 0;

accel = zeros(2,1);
steer = zeros(4,1);

% depending on the steering controller, either the 3 first or juste the
% last one will be filled.

%% Speed controller

Ts = 1/Fs;

% Converts desired speed into ref acceleration to get to that speed

% output acceleration (to be given to motor controller and it will do what
% it can)

% shaping controller, based on the error on speed. There is no feedback
% on acceleration yet
% the controller implemented is only proportional at the moment
a_ref_raw = low_ctr.K_accel * (v_ref - v) / Ts;

% saturation
a_ref = clip_signal(a_ref_raw, -low_ctr.max_accel, low_ctr.max_accel);


% TO IMPLEMENT LATER
% actual feedback loop on acceleration


%% Steering angle controller


% Angle steering ----------------
if steer_flag == 0;

    % shaping controller
    steer_ref = gamma_ref * steer_coeff;

    % feedback controller 
    % (not needed in this mode if we have a perfect mapping)
    steer_ref_fbk = steer_ref;

    % output
    steer_angle = steer_ref_fbk;


% Torque steering ----------------
elseif steer_flag == 1
    % only feedback for this one.

    % NOT IMPLEMENTED YET

end


%% Conversion of outputs

% accel to torque at wheels
torque_ref = mass * R_wheel * a_ref;

% gas pedal output
% torque at wheels to torque at engine (division by gear ratio)
torque_mot_ref = torque_ref / vhcl.gear_ratio;
% takes positive part of reference torque
gas_torque = clip_signal(torque_mot_ref, 0, inf);
% norms it with gas pedal to acceleration torque mapping
gas_out = gas_torque * torque_to_gas;
% clips to 1 (gas output is in [0;1])
gas_out_clipped = clip_signal(gas_out, 0, 1);

% brake pedal output
% takes negative part of reference torque and puts it in positive domain
% this is the TOTAL brake torque  at the wheels (sum on 4 wheels)
brake_torque = clip_signal(-torque_ref, 0, inf);
% norms it with gas pedal to acceleration torque mapping
% adds the two coeffs for each axle to be multiplied with the total torque
brake_out = brake_torque * sum(torque_to_brake);
% clips to 1 (brake output is in [0;1])
brake_out_clipped = clip_signal(brake_out, 0, 1);


%% Formatting of the outputs
% defines all bus variables for car control : gas/brake, lights, 
% blinkers, ... 

%
gas = gas_out_clipped;
brake = brake_out_clipped;


accel(1) = brake;
accel(2) = gas;

steer(1) = steer_angle;
steer(2) = steer_vel;
steer(3) = steer_acc;
steer(4) = steer_torque;


end



function x_clipped = clip_signal(x, lower_bnd, upper_bnd)
%%
%

x_clipped = max(lower_bnd, min(upper_bnd, x));

end

== matlab function cm_test/CarMaker/VehicleControl/Autonomous driving/trajectory tracking controller ==
  data: sensors_in input; v output; ctr_law input; vehicle input; gamma output; ctr_vars output
function [v, gamma, ctr_vars] = control_law(sensors_in, ctr_law, vehicle)
% input: "sensor_in", with the accessible fields:
% - imu_out
% - lat_errs
% - steer_angles
%
% fields of "sensors_in.imu_out" :
% - Omega_0 : gyro output on 3 axis in rad/s
% - Alpha_0 : accelerometers output on 3 
%
% fields of "lat_errs" :
% - lat_pos_ctr_road : 
% - lat_pos_ctr_lane :
% - hdg_err :
% - path_hdg :
% - curve_xy :
%
% fields of "steer_angles"
% - steer_angle_1 :
% - steer_angle_2 : 
% - mean_angle :

%% input retrieval


%% choice and application of control law

% markers for choosing the control law
Vilca_flag = ctr_law.flag == 1;
Stanley_flag = ctr_law.flag == 2;
Kinematic_flag = ctr_law.flag == 3;

if Vilca_flag
    % one term for the steering output has been deactivated
    [v, gamma, ctr_vars] = VilcaController(sensors_in, ctr_law, vehicle);
elseif Stanley_flag
    % Stanley's controller
    % NB; v is equal to the target speed specified in the parameters file.
    % This controller is not a speed controller.
    [v, gamma, ctr_vars] = StanleyController(sensors_in,...
        ctr_law, vehicle);
elseif Stanley_flag
    % Kinematic controller based on chained form
    [v, gamma, ctr_vars] = KinematicController(sensors_in, ctr_law, ...
        vehicle);
else
    v = 0;
    gamma = 0;
    ctr_vars = zeros(4,1);
end




end


function [v,gamma, ctr_vars] = ...
    VilcaController(sensors_in, ctr_law, vehicle)
%%
%

%% Control variables calculation

% target orientation in Fr0
% theta_T = sensors_in.rpsensor_out.path_hdg;

% angular error between vehicle direction and target direction
% DEBUG : "-" for correction of conventions
e_theta = - sensors_in(1).rpsensor_out.hdg_err;

% preview point pos wrt centre of rear axle
prev_pt_pos_r_axle = sensors_in(1).rpsensor_out.preview_pt_pos_Fr1 ...
    - [vehicle.rear_axle_x; 0; 0];
% x coordinate of target in Fr1 with rear axle as origin
e_x = prev_pt_pos_r_axle(1);
% y coordinate of target in Fr1 with rear axle as origin
e_y = prev_pt_pos_r_axle(2);
% absolute distance to target (preview point)
d = sqrt(e_x^2 + e_y^2);
% vehicle angular pos in target frame with reference direction being the
% direction of target but looking backwards
% is also:
% target heading - vehicle polar position in global frame as seen from
% target
% equation 3.13 of [Vilca2015]. The advantage is that it uses previously
% defined variables so if these ones are correct, the rest will also be.
e_RT = atan2(e_x*tan(e_theta)-e_y, e_x+tan(e_theta)*e_y);

% radius of curvature at target
r_ct = 1 / sensors_in(1).rpsensor_out.curve_xy; % careful if infinity
% target speed
% (projection of vehicle speed along path)
% in reality it's not ctr_law.target_speed because there will be a tracking
% error. The actual speed of the vehicle should be measured and projected
% on the path direction at the preview point
v_t = ctr_law.target_speed;
% pos of target in vehicle's frame


%% Parameters retrieval

% control law coeffs
% K_vec = zeros(1,6);
K_vec =  ctr_law.K_vilca;

K_d = K_vec(1);
K_l = K_vec(2);
K_o = K_vec(3);
K_x = K_vec(4);
K_RT = K_vec(5);
K_theta = K_vec(6);

% wheelbase
l_b = vehicle.wheelbase;

%% Pre-calculations

% CAUTION: the term with d^2 messes everything up. It is much bigger than
% the rest and leads to saturation.
c_c = 1 / (r_ct*cos(e_theta)) ...
    + K_theta * tan(e_theta) ...
    + ( K_d*e_y - K_l*d*sin(e_RT)*cos(e_theta) ) / (K_o*cos(e_theta)) ...
    + K_RT * sin(e_RT)^2 / (sin(e_theta)*cos(e_theta)) ; %...
%     + d^2*K_l*sin(e_RT)*cos(e_RT) / (r_ct*K_o*sin(e_theta)*cos(e_theta));

v_b = K_x * (   K_d*e_x ...
              + K_l*d*sin(e_RT)*sin(e_theta) ...
              + K_o*sin(e_theta)*c_c  );
          
%% Control variables output

ctr_vars = [e_x; 
            e_y; 
            e_theta; 
            e_RT];


%% Control law outputs

% speed output
v_raw = v_t * cos(e_theta) + v_b;

% steering output (rad)
gamma_raw = atan(l_b * c_c);
% gamma_raw = 0; % DEBUG

% saturation
v = clip_signal(v_raw, ctr_law.v_min, ctr_law.v_max);
gamma = clip_signal(gamma_raw, -ctr_law.gamma_max, ctr_law.gamma_max);


% debug point if saturation
if (v ~= v_raw) || (gamma ~= gamma_raw) || (abs(e_y) > 1e-1)
    0;
end

end


function [v,gamma, ctr_vars] = ...
    StanleyController(sensors_in, ctr_law, vehicle)
%%
% needs the prev point to be approx one car length forward (lateral info at
% front axle)

%% Parameters retrieval

% preview point pos wrt centre of front axle
prev_pt_pos_f_axle = sensors_in(1).rpsensor_out.preview_pt_pos_Fr1 ...
    - [vehicle.front_axle_x; 0; 0];

% control coefficients retrieval
K_stanley =  ctr_law.K_stanley;
k_main = K_stanley(1);
k_d_yaw = K_stanley(2);
k_soft = K_stanley(3);
k_d_steer = K_stanley(4);

%% Control parameters calculation

% angular error of vehicle traj wrt to path orientation
% it is the "e_theta" in the Vilca controller
% beware of sign conventions
psi = - sensors_in(1).rpsensor_out.hdg_err;

% actual speed
% the data is taken from the odometry (no GPS)
v_meas = sensors_in(1).odo_out.vel_from_motor;

% lateral error
e_y = prev_pt_pos_f_axle(2);

% car yaw rate
z_dot_car = sensors_in(1).imu_out.Omega_0(3);

% trajectory yaw rate
% curve * speed of preview point (car speed projected on trajectory)
z_dot_traj = sensors_in(1).rpsensor_out.curve_xy * v_meas * cos(psi);

% actual measured steering angle
gamma_meas = sensors_in(1).steersensor_out.mean_angle;

% previous measured steering angle
gamma_meas_prev = sensors_in(2).steersensor_out.mean_angle;

%% Steering control law

% main term
main_term = psi + atan2(k_main*e_y, v_meas + k_soft);

% yaw damping term for high speed instabilities
% WARNING: has strange effects with angle steering mode (because the
% steering is always infinitely fast in CarMaker)
yaw_damping_term = k_d_yaw * (z_dot_car - z_dot_traj);

% steering action damping (to account for delays in the actuation)
% WARNING : same as before
% WARNING 2 : sensitive to noise on steering angle measurement
steer_damping_term = k_d_steer * (gamma_meas - gamma_meas_prev);

% the steady state slip term has not been implemented yet.

%% Control variables output

ctr_vars = [main_term; % e_x wrt target (none here)
            e_y; 
            psi; % equivalent of e_theta in VilcaController 
            steer_damping_term]; % e_RT (none here)


%% Control law outputs

% does not control the speed, so just passes through the target
% (a speed controller is in fact evocated in the paper but it takes place
% at a low level. Thus it's just been used in a way to design our own
% speed controller).
v_raw = ctr_law.target_speed;

% raw steering angle (not clipped)
gamma_raw =   main_term ...         % ToDo : add other terms
            + yaw_damping_term...
            + steer_damping_term; 


% output signals
v = clip_signal(v_raw, ctr_law.v_min, ctr_law.v_max);
gamma = clip_signal(gamma_raw, -ctr_law.gamma_max, ctr_law.gamma_max);

end


function [v, gamma, ctr_vars] = ...
    KinematicController(sensors_in, ctr_law, vehicle)
%%
%
%
%

%% Parameters retrieval

% tuning coeff
k = ctr_law.K_kin;

% re-calculates the three coeffs for the ctrl law
k_1 = k^3;
k_2 = 3*k^2;
k_3 = 3*k;

% wheelbase
L = vehicle.wheelbase;

%% Control parameters calculation

% preview point pos wrt centre of rear axle (in Fr1)
preview_pt_pos_r_axle = sensors_in(1).rpsensor_out.preview_pt_pos_Fr1 ...
    - [vehicle.rear_axle_x; 0; 0];
preview_pt_pos_r_axle_prev = ...
    sensors_in(2).rpsensor_out.preview_pt_pos_Fr1 ...
    - [vehicle.rear_axle_x; 0; 0];
% lateral error
e_y = preview_pt_pos_r_axle(2); % "e_ra" in the paper
e_y_prev = preview_pt_pos_r_axle_prev(2);
% curvilinear position along path
s = sensors_in(1).rpsensor_out.s;
s_prev = sensors_in(2).rpsensor_out.s;
% curvature "K(s)"
curv = sensors_in(1).rpsensor_out.curve_xy;
curv_prev = sensors_in(2).rpsensor_out.curve_xy;
curv_pprev = sensors_in(3).rpsensor_out.curve_xy;
% derivative of curvature
curv_dot = (curv - curv_prev) * ctr_law.Fs;
curv_dot_prev = (curv_prev - curv_pprev) * ctr_law.Fs;
% angular error of vehicle traj wrt to path orientation
% it is the "e_theta" in the Vilca controller
% beware of sign conventions (different in each paper...)
theta_e = - sensors_in(1).rpsensor_out.hdg_err;
theta_e_prev = - sensors_in(2).rpsensor_out.hdg_err;
% measured steering angle
gamma_meas = sensors_in(1).steersensor_out.mean_angle;
gamma_meas_prev = sensors_in(2).steersensor_out.mean_angle;
% actual speed
% the data is taken from the odometry (no GPS)
v_meas = sensors_in(1).odo_out.vel_from_motor;

%% Change of coordinates for chained form

% practical coeff for future calculations
pcoeff = (1-e_y*curv) / cos(theta_e);

% new states
% x_1 = s; % curvilinear coord, we do not care here
x_2 = compute_x2(e_y, curv, curv_dot, theta_e, gamma_meas, L);
x_3 = pcoeff * sin(theta_e);
x_4 = e_y;

% new speed related input
u_1 = v_meas / pcoeff;

% re-ordering
X_2 = x_4;
X_3 = x_3;
X_4 = x_2;

%% Computes control law output with new states

u_2 = - k_1 * abs(u_1) * X_2 ...
      - k_2 * u_1 * X_3 ...
      - k_3 * abs(u_1) * X_4;

%% Go back to steering input from modified states/inputs

% need to compute:
% d(x_2)/d(s)
% d(x_2)/d(e_ra) (reminder: "e_ra" of the paper is "e_y" in the code)
% d(x_2)/d(theta_e)
%
% => need the previous: x_2, computed with previous: curv, curv_dot, e_y,
% theta_e, gamma_meas
% also need the previous: s, e_ra to compute ds, d(e_ra) and d(theta_e)

% computes previous x_2 state
x_2_prev = compute_x2(e_y_prev, curv_prev, curv_dot_prev, theta_e_prev, ...
            gamma_meas_prev, L);

% computes differences ("deltas")
delta_x_2 = x_2 - x_2_prev;
delta_s = s - s_prev;
delta_e_y = e_y - e_y_prev;
delta_theta_e = theta_e - theta_e_prev;

% computes coeffs for input transformation
% alpha_1
alpha_1 = delta_x_2 / delta_s ...
    + delta_x_2 / delta_e_y * pcoeff * sin(theta_e) ...
    + delta_x_2 / delta_theta_e * (pcoeff * tan(gamma_meas) / L - curv);
% alpha_2
alpha_2 = L * cos(gamma_meas)^2 * cos(theta_e) / pcoeff^2;

% computes the steering output (speed, not angle)
gamma_dot = alpha_2* ( u_2 - alpha_1*u_1 );

%% output

% converts steering speed into position (simple integration on sampling
% time)
gamma_raw = gamma_meas + gamma_dot / ctr_law.Fs;

% passes through desired speed
% a better speed controller/planner could be inserted here
v_raw = ctr_law.target_speed;

% clipping
v = clip_signal(v_raw, ctr_law.v_min, ctr_law.v_max);
gamma = clip_signal(gamma_raw, -ctr_law.gamma_max, ctr_law.gamma_max);

% control variables to monitor (unused for the moment)
ctr_vars = zeros(4,1);

end

function x_2 = compute_x2(e_y, curv, curv_dot, theta_e, gamma_meas, L)
%% calculation of x_2 state for kinematic controller
%

% practical calculation coeff
pcoeff = (1-e_y*curv) / cos(theta_e);

% new states
% x_1 = s; % curvilinear coord, we do not care here
x_2 = - curv_dot*e_y*tan(theta_e) ...
      - curv * pcoeff * (1+sin(theta_e)^2)/cos(theta_e) ...
      + pcoeff^2 * tan(gamma_meas) / (L*cos(theta_e));
  
end

function x_clipped = clip_signal(x, lower_bnd, upper_bnd)
%%
%

x_clipped = max(lower_bnd, min(upper_bnd, x));

end
